simulink model "APE_Project_Open Loop With Resitor_Buck"  (R2025a)
settings: Solver=VariableStepAuto  StartTime=0.0  StopTime=0.2  RelTol=1e-3
libraries: spsCurrentMeasurementLib x5, spsMosfetLib x4, spsSeriesRLCBranchLib x4, spsVoltageMeasurementLib x3, spsDCVoltageSourceLib x1, spsGroundLib x1, sps_lib x1
settings Model: Creator=KAILASH  LastModifiedBy=KAILASH

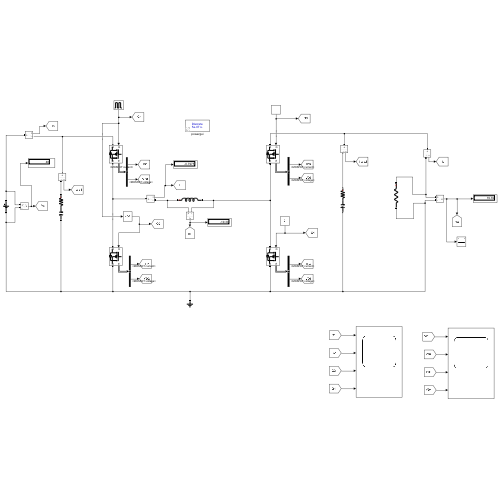
[thumbnail: Simulink's stored preview of the top-level diagram]
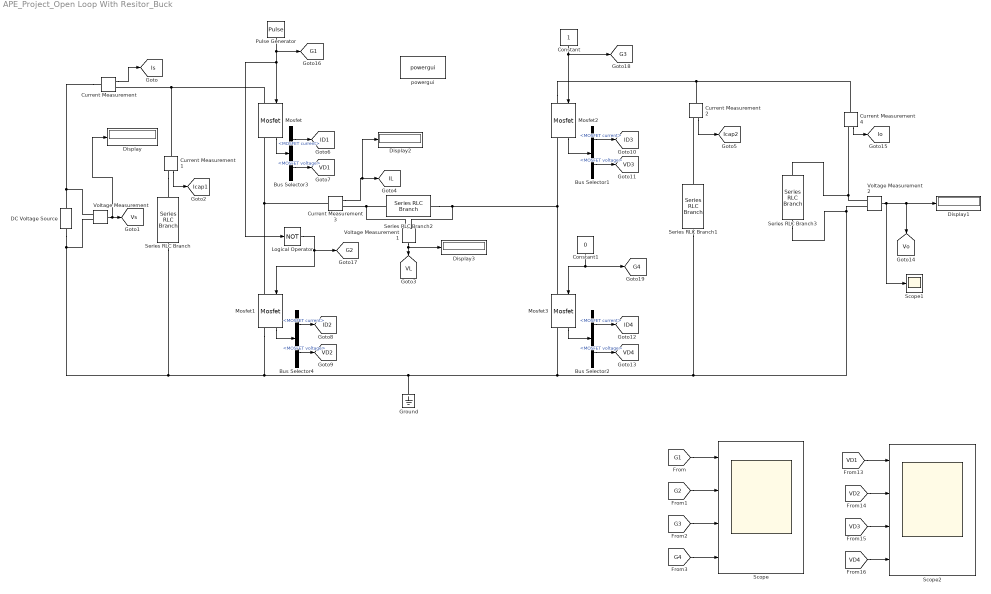
== system APE_Project_Open Loop With Resitor_Buck ==
  Bus Selector{1..4} (4 alike) : BusSelector  OutputSignals=MOSFET current,MOSFET voltage
  Constant : Constant
  Constant1 : Constant  Value=0
  Current Measurement{,1..4} (5 alike) : spsCurrentMeasurementLib/Current Measurement  PhasorSimulation=off  OutputType=Complex  PSBequivalent=0
  DC Voltage Source : spsDCVoltageSourceLib/DC Voltage Source  Amplitude=48  Measurements=Voltage
  Display{,1..3} (4 alike) : Display
  Ground : spsGroundLib/Ground  LConnTagsString=a
  Logical Operator : Logic  Operator=NOT  AllPortsSameDT=off  OutDataTypeStr=boolean
  Mosfet{,1..3} (4 alike) : spsMosfetLib/Mosfet  Ron=0.001  Lon=0  Rd=0.01  Vfd=0.8  IC=0  Rs=1e5  Cs=inf  Measurements=on
  Pulse Generator : DiscretePulseGenerator  PulseType=Time based  Period=1/75e3  PulseWidth=40
  Scope : Scope  NumInputPorts=4
      settings: ActiveDisplayYMinimum=-0.12499999999999997  ActiveDisplayYMaximum=1.125
  Scope1 : Scope
      settings: ActiveDisplayYMinimum=-5.933607269444491  ActiveDisplayYMaximum=53.522374292761612
  Scope2 : Scope  NumInputPorts=4
      settings: ActiveDisplayYMinimum=-6.0661334911892268  ActiveDisplayYMaximum=53.103619538638981  DataLoggingVariableName=ScopeData2
  Series RLC Branch : spsSeriesRLCBranchLib/Series RLC Branch  LConnTagsString=__new0  RConnTagsString=__new0  BranchType=RC  Resistance=0.001  Inductance=1e-3  SetiL0=off  InitialCurrent=0  Capacitance=488e-6  Setx0=off  InitialVoltage=48  Measurements=None
  Series RLC Branch1 : spsSeriesRLCBranchLib/Series RLC Branch  LConnTagsString=__new0  RConnTagsString=__new0  BranchType=RC  Resistance=0.001  Inductance=1e-3  SetiL0=off  InitialCurrent=0  Capacitance=488e-6  Setx0=off  InitialVoltage=36  Measurements=None
  Series RLC Branch2 : spsSeriesRLCBranchLib/Series RLC Branch  LConnTagsString=__new0  RConnTagsString=__new0  BranchType=L  Resistance=1  Inductance=150e-6  SetiL0=on  InitialCurrent=0  Capacitance=1e-6  Setx0=off  InitialVoltage=0  Measurements=None
  Series RLC Branch3 : spsSeriesRLCBranchLib/Series RLC Branch  LConnTagsString=__new0  RConnTagsString=__new0  BranchType=R  Resistance=100  Inductance=1e-3  SetiL0=off  InitialCurrent=0  Capacitance=1e-6  Setx0=off  InitialVoltage=0  Measurements=None
  Voltage Measurement : spsVoltageMeasurementLib/Voltage Measurement  PhasorSimulation=off  OutputType=Complex  PSBequivalent=0
  Voltage Measurement1 : spsVoltageMeasurementLib/Voltage Measurement  PhasorSimulation=off  OutputType=Complex  PSBequivalent=0
  Voltage Measurement2 : spsVoltageMeasurementLib/Voltage Measurement  PhasorSimulation=off  OutputType=Complex  PSBequivalent=0
  powergui : sps_lib/powergui  Priority=1  SimulationMode=Discrete  SampleTime=5e-7  frequency=60  Iterations=50  frequencyindice=0  Pbase=100e6  ErrMax=1e-4  UnitsV=kV  UnitsW=MW  buscounter=0  FunctionMessages=off  echomessages=off  EnableUseOfTLC=off  CurrentSourceSwitches=off  DisableSnubberDevices=off  DisableRonSwitches=off  DisableVfSwitches=off  DisplayEquations=off  AutomaticDiscreteSolvers=off  SolverType=Tustin/Backward Euler (TBE)  Interpol=off  ExternalGateDelay=off  methode=off  Ts=100  x0status=blocks  SPID=on  SwTol=0  HookPort=off  NonlinearTolerance=1e-4  nMaxIteration=100  ContinueOnMaxIteration=off  RestoreLinks=warning  ResistiveCurrentMeasurement=off  Frange=[0:2:500]  Ylog=off  Xlog=on  ShowGrid=off  save=off  variable=ZData  structure=0  ZoomFFT=off  StartTime=0.0  cycles=1  DisplayStyle=1  fundamental=60  FreqAxis=off  MaxFrequency=1000  frequencyindicesteady=1  RmsSteady=1  display=off
  tag scope: G1=global, G2=global, G3=global, G4=global, ID1=global, ID2=global, ID3=global, ID4=global, IL=global, Icap1=global, Icap2=global, Io=global, Is=global, VD1=global, VD2=global, VD3=global, VD4=global, VL=global, Vo=global, Vs=global
  wires:
  [G2] -> Scope/2
  Constant/1 -> [G3], Mosfet2/1
  Constant1/1 -> [G4], Mosfet3/1
  [G3] -> Scope/3
  [G4] -> Scope/4
  Pulse Generator/1 -> [G1], Mosfet/1, Logical Operator/1
  Bus Selector3/1 -> [ID1]  "<MOSFET current>"
  Current Measurement2/1 -> [Icap2]
  Voltage Measurement1/1 -> Display3/1, [VL]
  Bus Selector2/2 -> [VD4]  "<MOSFET voltage>"
  [VD1] -> Scope2/1
  Mosfet2/1 -> Bus Selector1/1
  Current Measurement3/1 -> Display2/1, [IL]
  Bus Selector1/2 -> [VD3]  "<MOSFET voltage>"
  [VD3] -> Scope2/3
  Mosfet/1 -> Bus Selector3/1
  Mosfet3/1 -> Bus Selector2/1
  Current Measurement4/1 -> [Io]
  Bus Selector4/1 -> [ID2]  "<MOSFET current>"
  Current Measurement1/1 -> [Icap1]
  [VD2] -> Scope2/2
  Current Measurement/1 -> [Is]
  Bus Selector4/2 -> [VD2]  "<MOSFET voltage>"
  [VD4] -> Scope2/4
  Mosfet1/1 -> Bus Selector4/1
  Bus Selector1/1 -> [ID3]  "<MOSFET current>"
  Bus Selector3/2 -> [VD1]  "<MOSFET voltage>"
  [G1] -> Scope/1
  Voltage Measurement/1 -> Display/1, [Vs]
  Logical Operator/1 -> [G2], Mosfet1/1
  Bus Selector2/1 -> [ID4]  "<MOSFET current>"
  Voltage Measurement2/1 -> Scope1/1, [Vo], Display1/1
  connections:
  Current Measurement3/RConn1 -- Series RLC Branch2/LConn1 -- Voltage Measurement1/LConn1
  Current Measurement/RConn1 -- Mosfet/LConn1 -- Current Measurement1/LConn1
  Mosfet2/LConn1 -- Current Measurement2/LConn1 -- Current Measurement4/LConn1
  Series RLC Branch3/RConn1 -- Voltage Measurement2/LConn2 -- Series RLC Branch1/RConn1 -- Ground/LConn1 -- Mosfet1/RConn1 -- Series RLC Branch/RConn1 -- Voltage Measurement/LConn2 -- DC Voltage Source/LConn1 -- Mosfet3/RConn1
  Current Measurement/LConn1 -- DC Voltage Source/RConn1 -- Voltage Measurement/LConn1
  Mosfet2/RConn1 -- Mosfet3/LConn1 -- Voltage Measurement1/LConn2 -- Series RLC Branch2/RConn1
  Mosfet/RConn1 -- Mosfet1/LConn1 -- Current Measurement3/LConn1
  Current Measurement4/RConn1 -- Voltage Measurement2/LConn1 -- Series RLC Branch3/LConn1
  Current Measurement1/RConn1 -- Series RLC Branch/LConn1
  Series RLC Branch1/LConn1 -- Current Measurement2/RConn1
